simulink model "v2021_10_27_Density_height_SITL"  (R2018b)
settings: Solver=ode4  StartTime=0.0  StopTime=0  FixedStep=0.01  RelTol=1e-3
values from neighbouring files (symbols this model uses):
  h0 = input('inserire la quota desiderata: ')    [trimCalc.m]
libraries: aerolibatmos2 x1
settings Model: Creator=Giorgio  LastModifiedBy=Giorgio

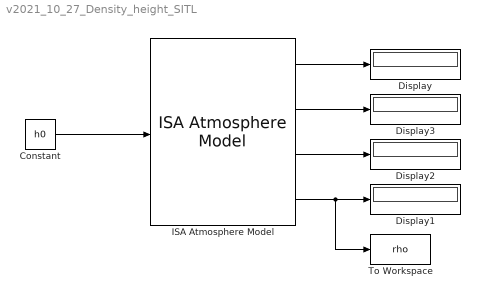
== system v2021_10_27_Density_height_SITL ==
  Constant : Constant  Value=h0
  Display{,1..3} (4 alike) : Display
  ISA Atmosphere Model : aerolibatmos2/ISA Atmosphere Model  custom=off  g=9.80665  gamma=1.4  R=287.0531  L=0.0065  h_trop=11000  h_strat=20000  rho0=1.225  P0=101325  T0=288.15  h0=0
      settings: SourceProductName=Aerospace Blockset
  To Workspace : ToWorkspace  VariableName=rho  SampleTime=-1
  wires:
  Constant/1 -> ISA Atmosphere Model/1
  ISA Atmosphere Model/1 -> Display/1
  ISA Atmosphere Model/2 -> Display3/1
  ISA Atmosphere Model/3 -> Display2/1
  ISA Atmosphere Model/4 -> To Workspace/1, Display1/1
